simulink model "stellaris_lp_irreceive_ROOMBA"  (R2017a)
settings: Solver=ode3  StartTime=0.0  StopTime=0.5  FixedStep=0.0002  RelTol=1e-3
values from neighbouring files (symbols this model uses):
  bits = [bits 0]    [stellaris_lp_irreceive_setup.m]
libraries: stellaris_lp_lib x4, simulink x3
settings Model: ExtModeTrigDuration=2  Creator=peselnikmg  LastModifiedBy=Nilim
settings DataIOCC: LimitDataPoints=on  SaveFormat=Array  SignalLoggingSaveFormat=ModelDataLogs
settings OptimizationCC: PassReuseOutputArgsAs=Individual arguments  ExpressionDepthLimit=2147483647  MaxStackSize=64
settings DebuggingCC: UnderspecifiedInitializationDetection=Classic  MergeDetectMultiDrivingBlocksExec=none  ParameterTunabilityLossMsg=error  StateNameClashWarn=warning  SFUnexpectedBacktrackingDiag=warning  SFNoUnconditionalDefaultTransitionDiag=warning  SFExecutionAtInitializationDiag=none
settings HardwareCC: ProdBitPerPointer=32  ProdBitPerSizeT=32  ProdBitPerPtrDiffT=32  ProdLargestAtomicInteger=Long  ProdLargestAtomicFloat=Double  ProdWordSize=32  ProdHWDeviceType=ARM Compatible->ARM Cortex
settings ModelReferenceCC: PropagateSignalLabelsOutOfModel=off
settings SFSimCC: MATLABDynamicMemAlloc=off
settings RTWCC: SystemTargetFile=ert.tlc  HardwareBoard=Tiva TM4C123G Launchpad  TLCOptions=-aInlineSetEventsForThisBaseRateFcn=TLC_FALSE -aSuppressMultiTaskScheduler=TLC_FALSE -aRateBasedStepFcn=1  TemplateMakefile=ert_default_tmf  Description=Embedded Coder  GenerateReport=on  RTWVerbose=off  Toolchain=Texas Instruments Code Composer Studio (Tiva)  IncludeHyperlinkInReport=on  LaunchReport=on  GenerateTraceInfo=on  GenerateTraceReport=on  GenerateTraceReportSl=on  GenerateTraceReportSf=on  GenerateTraceReportEml=on
settings CodeAppCC: ForceParamTrailComments=on  IgnoreCustomStorageClasses=off  OperatorAnnotations=on  SimulinkDataObjDesc=on  SFDataObjDesc=on  MATLABFcnDesc=on  CustomSymbolStrType=$N$R$M  InsertBlockDesc=on  MATLABSourceComments=on  InternalIdentifier=Classic
settings ConfigComp: CovMetricSettings=dw  CovHtmlReporting=on  CovSaveCumulativeToWorkspaceVar=on  CovSaveSingleToWorkspaceVar=on  CovExternalEMLEnable=off

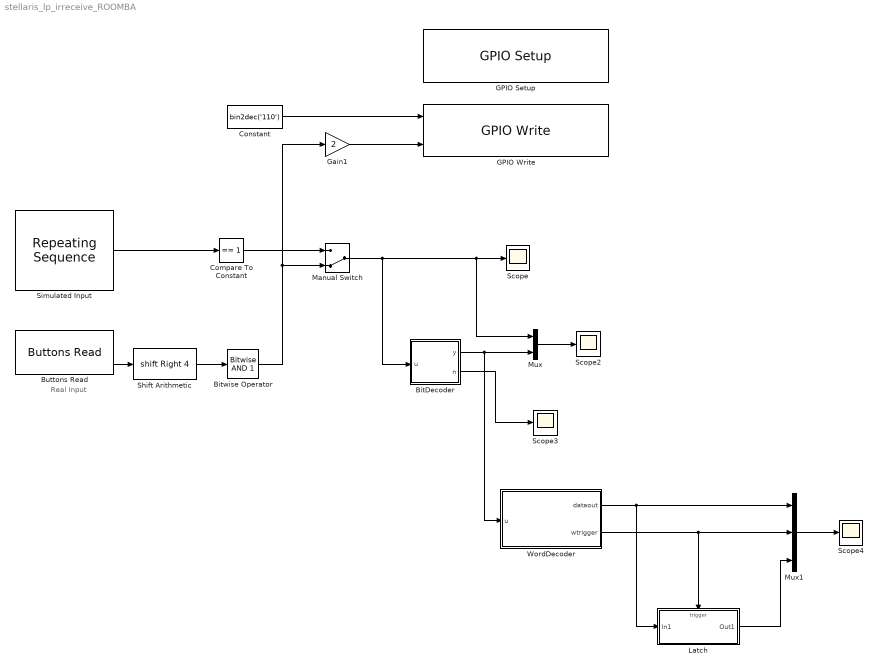
== system stellaris_lp_irreceive_ROOMBA ==
  note: Real Input
  BitDecoder : Stateflow chart  TreatAsAtomicUnit=on
  Bitwise Operator : simulink/Logic and Bit Operations/Bitwise Operator  logicop=AND  UseBitMask=on  BitMask=1  BitMaskRealWorld=Stored Integer
  Buttons Read : stellaris_lp_lib/Buttons/Buttons Read  SampleTime=-1
      settings: SourceProductName=Run on Stellaris LaunchPad
  Compare To Constant : simulink/Logic and Bit Operations/Compare To Constant  relop===  const=1  OutDataTypeStr=uint8
  Constant : Constant  Value=bin2dec('110')  OutDataTypeStr=Inherit: Inherit via back propagation
  GPIO Setup : stellaris_lp_lib/GPIO/GPIO Setup  GPIO_PORTX_BASE=GPIO_PORTF_BASE  PinsOutput_0=Input  PinsOutput_1=Output  PinsOutput_2=Output  PinsOutput_3=Output  PinsOutput_4=Input  PinsOutput_5=Input  PinsOutput_6=Input  PinsOutput_7=Input
      settings: SourceProductName=Run on Stellaris LaunchPad
  GPIO Write : stellaris_lp_lib/GPIO/GPIO Write  GPIO_PORTX_BASE=GPIO_PORTF_BASE  SampleTime=-1
      settings: SourceProductName=Run on Stellaris LaunchPad
  Gain1 : Gain  Gain=2  OutDataTypeStr=Inherit: Inherit via back propagation
  Latch : Subsystem  TreatAsAtomicUnit=on
  Manual Switch : ManualSwitch  CurrentSetting=0
  Mux : Mux  Inputs=2
  Mux1 : Mux  Inputs=3
  Scope{,2..4} (4 alike) : Scope
  Shift Arithmetic : ArithShift  BitShiftNumber=4  BitShiftDirection=Right
  Simulated Input : simulink/Sources/Repeating Sequence  rep_seq_t=bitt  rep_seq_y=int32(bits)
  WordDecoder : Stateflow chart  TreatAsAtomicUnit=on
  wires:
  Simulated Input/1 -> Compare To Constant/1
  Manual Switch/1 -> Mux/1, Scope/1, BitDecoder/1(u)
  Mux/1 -> Scope2/1
  BitDecoder/2(n) -> Scope3/1
  BitDecoder/1(y) -> WordDecoder/1(u), Mux/2
  Mux1/1 -> Scope4/1
  WordDecoder/1(dataout) -> Latch/1(In1), Mux1/1
  WordDecoder/2(wtrigger) -> Latch/Trigger, Mux1/2
  Compare To Constant/1 -> Manual Switch/1
  Buttons Read/2 -> Shift Arithmetic/1
  Latch/1(Out1) -> Mux1/3
  Constant/1 -> GPIO Write/1
  Gain1/1 -> GPIO Write/2
  Bitwise Operator/1 -> Gain1/1, Manual Switch/2
  Shift Arithmetic/1 -> Bitwise Operator/1

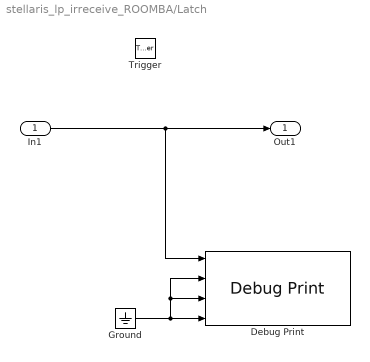
== system stellaris_lp_irreceive_ROOMBA/Latch ==
  In1 : Inport
  Trigger : TriggerPort  VariantControl=Variant
  Debug Print : stellaris_lp_lib/Debug/Debug Print  fmt='Got command %d'  sample_time=-1
      settings: SourceProductName=Run on Stellaris LaunchPad
  Ground : Ground
  Out1 : Outport
  wires:
  In1/1 -> Debug Print/1, Out1/1
  Ground/1 -> Debug Print/4, Debug Print/3, Debug Print/2

== stateflow chart stellaris_lp_irreceive_ROOMBA/BitDecoder ==
  state Start
    y=7;
    n=0;
  state WaitBit
    y=6;
    n=n+1;
    m=0;
  state GotBit0
    y=0;
    n=0;
    m=m+1;
  state GotBit1
    y=1;
    n=0;
    m=m+1;
  GotBit0 -> Start [order 3] : [u==0 && m>=30]
  GotBit0 -> WaitBit [order 2] : [u==1]
  (default) -> Start
  Start -> WaitBit : [u==1]
  WaitBit -> GotBit0 [order 1] : [u==0 && n<10]
  GotBit0 -> GotBit0 [order 1] : [u==0 && m<30]
  WaitBit -> GotBit1 [order 3] : [u==0 && n>=10]
  WaitBit -> WaitBit [order 2] : [u==1]
  GotBit1 -> Start [order 3] : [u==0 && m>=30]
  GotBit1 -> WaitBit [order 2] : [u==1]
  GotBit1 -> GotBit1 [order 1] : [u==0 && m<30]
  data: u input; y output int32; n output int32; m local int32

== stateflow chart stellaris_lp_irreceive_ROOMBA/WordDecoder ==
  state Start
    nb=0;
    data=0;
    dataout=0;
    wtrigger=0;
  state BitComing
  state GotBit
    nb=nb+1;
    data=data*2+u;
  state Output
    dataout=data;
    wtrigger=1;
  GotBit -> Start [order 2] : [u==7]
  GotBit -> BitComing [order 1] : [u==6]
  (default) -> Start
  BitComing -> GotBit : [u!=6]
  Start -> BitComing : [u==6]
  GotBit -> Output [order 3] : [nb==8]
  Output -> Start
  data: u input; dataout output int32; wtrigger output int32; data local int32; nb local int32
